simulink model "Simulation"  (R2023b)
settings: Solver=VariableStepAuto  StartTime=0.0  StopTime=20  RelTol=1e-3
undefined symbols (not defined in the file): A, B, C, D, data
libraries: SignalEditorBlockLib x1
settings Model: Creator=ematric  LastModifiedBy=fluky

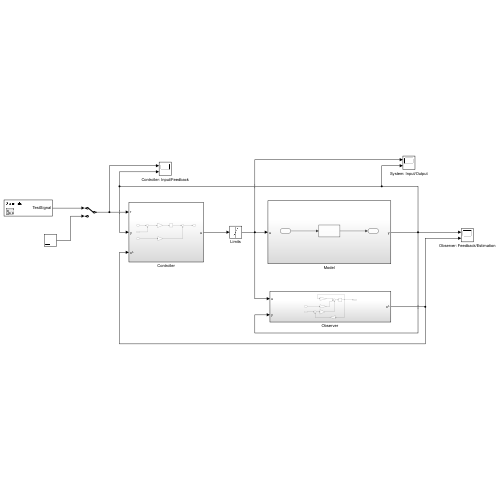
[thumbnail: Simulink's stored preview of the top-level diagram]
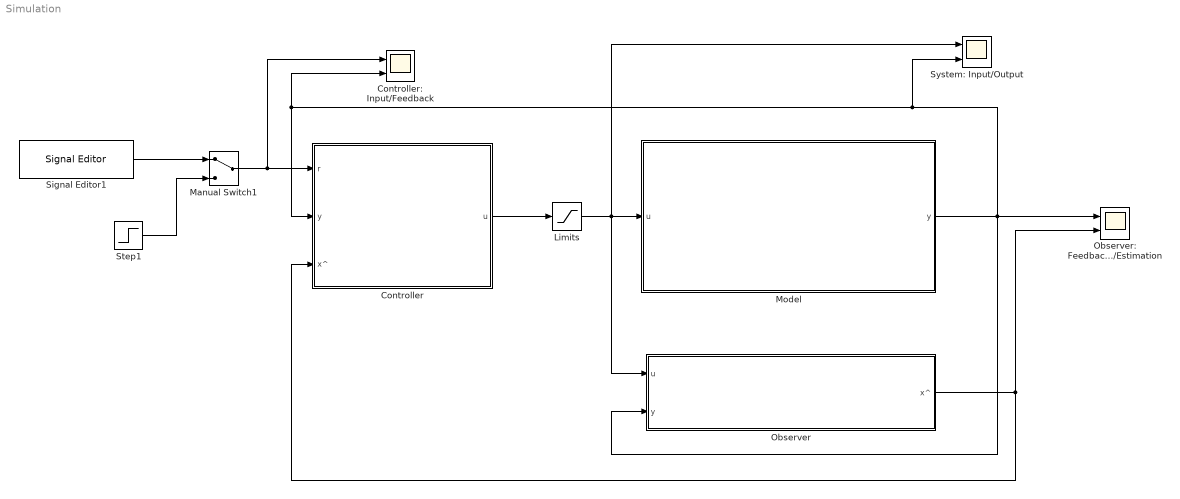
== system Simulation ==
  Controller : Subsystem
  Controller: Input/Feedback : Scope  NumInputPorts=2
  Limits : Saturate  UpperLimit=5  LowerLimit=-5
  Manual Switch1 : ManualSwitch
  Model : Subsystem
  "Observer " : Subsystem
  Observer: Feedback/Estimation : Scope  NumInputPorts=2
  Signal Editor1 : SignalEditorBlockLib/Signal Editor  FileName=C:\workspace\matlabControlLab\lab1 - Levitation\240113lab\240129preparation\trajectories.mat  ActiveScenario=Scenario  ActiveSignal=TestSignal  IsBus=off  OutputBusObjectStr=Bus: BusObject  SampleTime=0  Interpolate=off  ZeroCross=off  OutputAfterFinalValue=Setting to zero  Unit=inherit  PreserveSignalName=on  ApplySigPropsToAllScenarios=on  ApplySigPropsToAllSignals=off
  Step1 : Step  SampleTime=0
  System: Input/Output : Scope  NumInputPorts=2
  wires:
  Controller/1(u) -> Limits/1
  Limits/1 -> System: Input/Output/1, Model/1(u), "Observer "/1(u)
  Model/1(y) -> Observer: Feedback/Estimation/1, "Observer "/2(y), System: Input/Output/2, Controller/2(y), Controller: Input/Feedback/2
  "Observer "/1(x^) -> Controller/3(x^), Observer: Feedback/Estimation/2
  Signal Editor1/1 -> Manual Switch1/1
  Step1/1 -> Manual Switch1/2
  Manual Switch1/1 -> Controller: Input/Feedback/1, Controller/1(r)

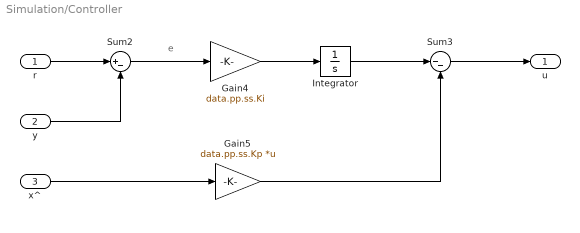
== system Simulation/Controller ==
  note: e
  r : Inport
  y : Inport  Port=2
  x^ : Inport  Port=3
  Gain4 : Gain  Gain=data.pp.ss.Ki
  Gain5 : Gain  Gain=data.pp.ss.Kp  Multiplication=Matrix(K*u)
  Integrator : Integrator
  Sum2 : Sum  Inputs=|+-
  Sum3 : Sum  Inputs=|--
  u : Outport
  wires:
  Integrator/1 -> Sum3/1
  Gain4/1 -> Integrator/1
  Sum2/1 -> Gain4/1
  Gain5/1 -> Sum3/2
  r/1 -> Sum2/1
  y/1 -> Sum2/2
  Sum3/1 -> u/1
  x^/1 -> Gain5/1

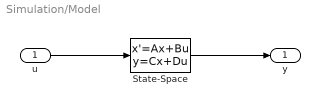
== system Simulation/Model ==
  u : Inport
  State-Space : StateSpace  A=A  B=B  C=C  D=D  InitialCondition=0
  y : Outport
  wires:
  u/1 -> State-Space/1
  State-Space/1 -> y/1

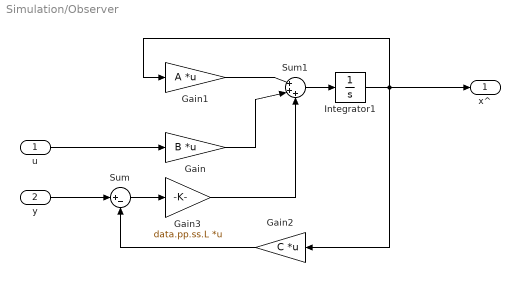
== system Simulation/Observer  ==
  u : Inport
  y : Inport  Port=2
  Gain : Gain  Gain=B  Multiplication=Matrix(K*u)
  Gain1 : Gain  Gain=A  Multiplication=Matrix(K*u)
  Gain2 : Gain  Gain=C  Multiplication=Matrix(K*u)
  Gain3 : Gain  Gain=data.pp.ss.L  Multiplication=Matrix(K*u)
  Integrator1 : Integrator
  Sum : Sum  Inputs=|+-
  Sum1 : Sum  Inputs=|+++
  x^ : Outport
  wires:
  Gain1/1 -> Sum1/1
  Gain2/1 -> Sum/2
  Sum/1 -> Gain3/1
  Integrator1/1 -> x^/1, Gain2/1, Gain1/1
  Gain/1 -> Sum1/2
  Gain3/1 -> Sum1/3
  Sum1/1 -> Integrator1/1
  u/1 -> Gain/1
  y/1 -> Sum/1
